simulink model "planta_controlador"  (R2025b)
settings: Solver=FixedStepAuto  StartTime=0.0  StopTime=inf  FixedStep=Ts2  MaxStep=1e-3  RelTol=1e-3
undefined symbols (not defined in the file): ah_max, at_max, bcx, bcy, bh_eq, bhb, bhEb, bhwu, bt, bt_eq, btb, btw, counter_limit, DiscIntNeverNeededParam, g, h_vec_inicial, Hc, ih, is_scanned_vec_inicial, it, Jh_eq, Jt_eq, Kcy, khwu, Ki_h, Ki_t, Kp_h, Kp_t, Ktw, lambda, Lh, Lh0, lh_0, Lt, magnitude, Mc_max, Ms, Mt, N_xt, P_nom, periodo_pulsos, rhd, rtd, tau_hm, tau_tm, Thb_Max, ThEb_Max, Thm_0, Thm_Max, titahm_0, titatm_0, Ts0, Ts1, Ts2, Ttb_Max, Ttm_0, Ttm_Max, vh_0, vh_max_unloaded, vh_nom ... (+20)
libraries: simulink x17, simulink_extras x2, sl3dlib x1, dspnetwork x1
(part 2 of 2)

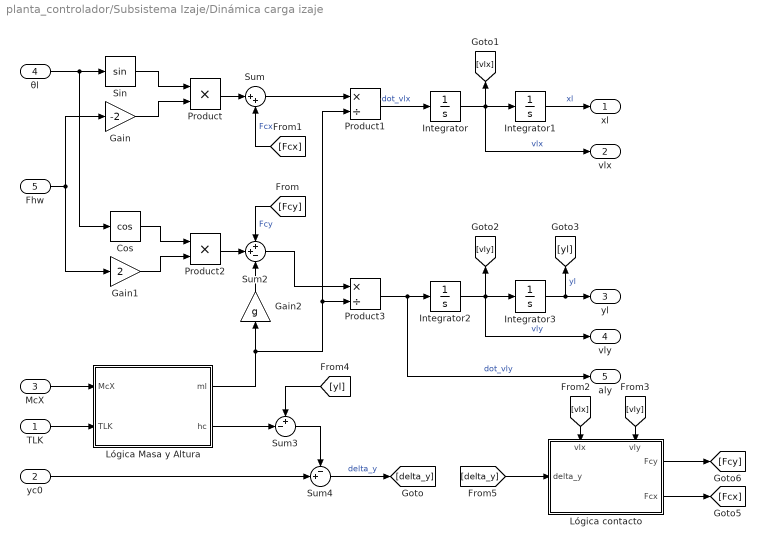
== system planta_controlador/Subsistema Izaje/Dinámica carga izaje ==
  TLK : Inport
  yc0 : Inport  Port=2
  McX : Inport  Port=3
  θl : Inport  Port=4
  Fhw : Inport  Port=5
  Cos : Trigonometry  Operator=cos
  Gain : Gain  Gain=-2
  Gain1 : Gain  Gain=2
  Gain2 : Gain  Gain=g
  Integrator : Integrator  InitialCondition=vlx_0
  Integrator1 : Integrator  InitialCondition=xl_0
  Integrator2 : Integrator  InitialCondition=vly_0
  Integrator3 : Integrator  InitialCondition=yl_0
  Lógica Masa y Altura : Subsystem
  Lógica contacto : Subsystem
      settings: PortSchema="{\"entries\":[{\"content\":{\"sides\":[{\"content\":{\"connectorIds\":[\"In1\"]},\"type\":\"ConnectorPlacement.EquallySpacedRectSide\",\"uuid\":\"20a8b2c4-d5cf-44ce-93ec-929b996a0905\"},{\"content\":{\"connectorIds\":[\"Out1\",\"Out2\"],\"side\":\"RIGHT\"},\"type\":\"ConnectorPlacement.EquallySpacedRectSide\",\"uuid\":\"396e1f2e-cf71-48dc-8d57-a3e2695dfff1\"},{\"content\":{\"connectorIds\":[\"In2\",\"In3\"],\"side\":\"TOP\"},\"type\":\"ConnectorPlacement.EquallySpacedRectSide\",\"uuid\":\"e66c0478-9682-41e1-9b77-d2d789a9c323\"}]},\"type\":\"ConnectorPlacement.EquallySpacedConnector\",\"uuid\":\"193dabd2-f524-433a-b6ef-c1cab585578e\"}],\"packageUris\":[\"http://schema.mathworks.com/mf0/Connector/R2020b\"],\"version\":\"1.0\"}"
  Product : Product
  Product1 : Product  Inputs=*/
  Product2 : Product
  Product3 : Product  Inputs=*/
  Sin : Trigonometry
  Sum : Sum  Inputs=|++
  Sum2 : Sum  Inputs=++-
  Sum3 : Sum  Inputs=+-|
  Sum4 : Sum  Inputs=-+|
  xl : Outport
  vlx : Outport  Port=2
  yl : Outport  Port=3
  vly : Outport  Port=4
  aly : Outport  Port=5
  wires:
  θl/1 -> Sin/1, Cos/1
  Integrator/1 -> vlx/1, Integrator1/1, [vlx]  "vlx"
  Sum3/1 -> Sum4/1
  Sin/1 -> Product/1
  Gain/1 -> Product/2
  [Fcy] -> Sum2/1  "Fcy"
  Integrator2/1 -> vly/1, Integrator3/1, [vly]  "vly"
  Integrator3/1 -> yl/1, [yl]  "yl"
  Fhw/1 -> Gain1/1, Gain/1
  [Fcx] -> Sum/2  "Fcx"
  Product/1 -> Sum/1
  Product1/1 -> Integrator/1  "dot_vlx"
  Gain2/1 -> Sum2/3
  Cos/1 -> Product2/1
  Gain1/1 -> Product2/2
  [yl] -> Sum3/1
  Product2/1 -> Sum2/2
  yc0/1 -> Sum4/2
  Sum2/1 -> Product3/1
  Product3/1 -> aly/1, Integrator2/1  "dot_vly"
  Sum/1 -> Product1/1
  Integrator1/1 -> xl/1  "xl"
  Sum4/1 -> [delta_y]  "delta_y"
  Lógica contacto/1(Fcy) -> [Fcy]
  Lógica contacto/2(Fcx) -> [Fcx]
  Lógica Masa y Altura/1(ml) -> Product1/2, Product3/2, Gain2/1
  McX/1 -> Lógica Masa y Altura/1(McX)
  TLK/1 -> Lógica Masa y Altura/2(TLK)
  Lógica Masa y Altura/2(hc) -> Sum3/2
  [vlx] -> Lógica contacto/2(vlx)
  [vly] -> Lógica contacto/3(vly)
  [delta_y] -> Lógica contacto/1(delta_y)

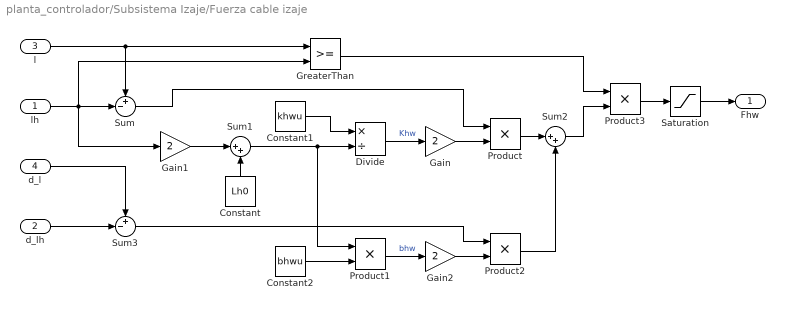
== system planta_controlador/Subsistema Izaje/Fuerza cable izaje ==
  lh : Inport
  d_lh : Inport  Port=2
  l : Inport  Port=3
  d_l : Inport  Port=4
  Constant : Constant  Value=Lh0
  Constant1 : Constant  Value=khwu
  Constant2 : Constant  Value=bhwu
  Divide : Product  Inputs=*/  RndMeth=Zero  SaturateOnIntegerOverflow=on
  Gain : Gain  Gain=2
  Gain1 : Gain  Gain=2
  Gain2 : Gain  Gain=2
  GreaterThan : RelationalOperator  OutDataTypeStr=boolean  RndMeth=Simplest  InputSameDT=off
  Product{,1..3} (4 alike) : Product
  Saturation : Saturate  UpperLimit=inf  LowerLimit=0
  Sum : Sum  Inputs=+-|
  Sum1 : Sum  Inputs=|++
  Sum2 : Sum  Inputs=|++
  Sum3 : Sum  Inputs=+-|
  Fhw : Outport
  wires:
  Constant/1 -> Sum1/2
  Constant2/1 -> Product1/2
  Sum1/1 -> Divide/2, Product1/1
  lh/1 -> Sum/2, GreaterThan/2, Gain1/1
  Product/1 -> Sum2/1
  Gain1/1 -> Sum1/1
  l/1 -> Sum/1, GreaterThan/1
  Product2/1 -> Sum2/2
  Product3/1 -> Saturation/1
  GreaterThan/1 -> Product3/1
  d_lh/1 -> Sum3/2
  Constant1/1 -> Divide/1
  Product1/1 -> Gain2/1  "bhw"
  Sum/1 -> Product/1
  Gain2/1 -> Product2/2
  Divide/1 -> Gain/1  "Khw"
  Sum2/1 -> Product3/2
  Sum3/1 -> Product2/1
  d_l/1 -> Sum3/1
  Gain/1 -> Product/2
  Saturation/1 -> Fhw/1

== system planta_controlador/Subsistema Carro/Accionamiento carro/Freno Motor ==
  BRK_t : Inport
  wtm : Inport  Port=2
  Constant : Constant  Value=0
  Gain3 : Gain  Gain=-Ttb_Max
  Gain4 : Gain  Gain=btb
  Switch : Switch  Criteria=u2 > Threshold  SaturateOnIntegerOverflow=off  InputSameDT=off
  Tanh : Trigonometry  Operator=tanh
  Ttb : Outport
  wires:
  BRK_t/1 -> Switch/2
  Constant/1 -> Switch/1
  wtm/1 -> Gain4/1
  Gain4/1 -> Tanh/1
  Tanh/1 -> Gain3/1
  Gain3/1 -> Switch/3
  Switch/1 -> Ttb/1

== system planta_controlador/Subsistema Izaje/Accionamiento izaje/Freno Emergencia (Drum) ==
  BRK_hE : Inport
  whd : Inport  Port=2
  Constant : Constant  Value=0
  Gain3 : Gain  Gain=-ThEb_Max
  Gain4 : Gain  Gain=bhEb
  Switch : Switch  Criteria=u2 > Threshold  SaturateOnIntegerOverflow=off  InputSameDT=off
  Tanh : Trigonometry  Operator=tanh
  ThEb : Outport
  wires:
  BRK_hE/1 -> Switch/2
  Gain3/1 -> Switch/3
  Constant/1 -> Switch/1
  whd/1 -> Gain4/1
  Gain4/1 -> Tanh/1
  Tanh/1 -> Gain3/1
  Switch/1 -> ThEb/1

== system planta_controlador/Subsistema Izaje/Accionamiento izaje/Freno Motor ==
  BRK_h : Inport
  whm : Inport  Port=2
  Constant : Constant  Value=0
  Gain3 : Gain  Gain=-Thb_Max
  Gain4 : Gain  Gain=bhb
  Switch : Switch  Criteria=u2 > Threshold  SaturateOnIntegerOverflow=off  InputSameDT=off
  Tanh : Trigonometry  Operator=tanh
  Thb : Outport
  wires:
  BRK_h/1 -> Switch/2
  Gain3/1 -> Switch/3
  Constant/1 -> Switch/1
  whm/1 -> Gain4/1
  Gain4/1 -> Tanh/1
  Tanh/1 -> Gain3/1
  Switch/1 -> Thb/1

== system planta_controlador/Subsistema Izaje/Dinámica carga izaje/Lógica Masa y Altura ==
  McX : Inport
  TLK : Inport  Port=2
  Constant : Constant  Value=Ms
  Constant1 : Constant  Value=0
  Constant2 : Constant  Value=Hc
  Rate Limiter : RateLimiter  Commented=through  RisingSlewLimit=Mc_max/0.1  FallingSlewLimit=-Mc_max/0.1  SampleTimeMode=inherited  InitialCondition=Ms
  Sum1 : Sum  Inputs=|++
  Switch : Switch  Criteria=u2 > Threshold  SaturateOnIntegerOverflow=off  InputSameDT=off
  Switch1 : Switch  Criteria=u2 > Threshold  SaturateOnIntegerOverflow=off  InputSameDT=off
  ml : Outport
  hc : Outport  Port=2
  wires:
  Sum1/1 -> Switch/1
  Constant2/1 -> Switch1/1
  TLK/1 -> Switch1/2, Switch/2
  Constant/1 -> Switch/3, Sum1/2
  Constant1/1 -> Switch1/3
  McX/1 -> Sum1/1
  Switch/1 -> Rate Limiter/1
  Rate Limiter/1 -> ml/1
  Switch1/1 -> hc/1

== system planta_controlador/Subsistema Izaje/Dinámica carga izaje/Lógica contacto ==
  delta_y : Inport
  vlx : Inport  Port=2
  vly : Inport  Port=3
  Constant3 : Constant  Value=0
  Constant4 : Constant  Value=0
  Gain3 : Gain  Gain=Kcy
  Gain4 : Gain  Gain=bcy
  Gain5 : Gain  Gain=-bcx
  Saturation : Saturate  UpperLimit=60e5  LowerLimit=0
  Sum5 : Sum  Inputs=-+|
  Switch2 : Switch  SaturateOnIntegerOverflow=off  InputSameDT=off
  Switch3 : Switch  SaturateOnIntegerOverflow=off  InputSameDT=off
  Fcy : Outport
  Fcx : Outport  Port=2
  wires:
  Sum5/1 -> Switch2/1
  vlx/1 -> Gain5/1
  Gain4/1 -> Sum5/1
  vly/1 -> Gain4/1
  Constant4/1 -> Switch3/3
  Gain5/1 -> Switch3/1
  Gain3/1 -> Sum5/2
  delta_y/1 -> Switch3/2, Gain3/1, Switch2/2
  Constant3/1 -> Switch2/3
  Switch2/1 -> Saturation/1  "Fcy"
  Switch3/1 -> Fcx/1  "Fcx"
  Saturation/1 -> Fcy/1

== matlab function planta_controlador/MATLAB Function ==
  data: TLK input; M_carga output; Mc_min parameter
function M_carga = Masa_Aleatoria(TLK, Mc_min)
    persistent masa_actual;
    persistent ultimo_estado_trigger;
    
    % Inicialización
    if isempty(masa_actual)
        masa_actual = Mc_min; % Empezamos con el valor mínimo por defecto
        ultimo_estado_trigger = 0;
    end
    
    % DETECCIÓN DE FLANCO DE SUBIDA (Rising Edge)
    if (TLK == 1 && ultimo_estado_trigger == 0)
        % Generar carga aleatoria entre 3tn y 55tn (para tener sobrecarga)
        masa_actual = Mc_min + (55000 - Mc_min) * rand();
        masa_actual = round(masa_actual); 
    end
    
    % Actualizar memoria del trigger
    ultimo_estado_trigger = TLK;
    % Salida: La masa se mantiene constante hasta el próximo trigger
    M_carga = masa_actual;
end

== stateflow chart planta_controlador/Control Nivel 1 ==
  settings: updateMethod=DISCRETE  sampleTime=Ts1
  state AUTOMATA_PRINCIPAL [parallel]
    entry:
    dead_zone = 0.1; % Zona muerta joystick
    modo_posicion_segura = 0;
    modo_manual_auto = 0;
    seleccionando = 0; ejec_mov = 0;
    is_cont = 0; seleccionando = 0;
    error_der = 0; error_izq = 0;
    error_sup = 0; error_inf = 0;
    error_generic = 0;
    envolvente = zeros(33,1);
    during:
    Joy_CMD_X = Joy_XY(1);
    Joy_CMD_Y = Joy_XY(2);
    settings: executionOrder=1
    state MODO_AUTO
      exit:
      seleccionando_i = [0,0];
      i_obj_vec = [0,0];
      modo_auto = 0;
      modo_manual_auto = 0;
      seleccionando = 0;
      ejec_mov = 0;
      state SELECCION_INDICE_INI
        entry:
        seleccionando_i(1) = 1;
        seleccionando = 1;
        during:
        i_ini = i_x_cruz;
        is_cont = Check_Container(i_ini, yc0_vec);
        exit:
        i_obj_vec(1) = i_ini;
        seleccionando_i(1) = 0;
      state SELECCION_INDICE_FIN
        entry:
        seleccionando_i(2) = 1;
        seleccionando = 1;
        invalido = 0;
        during:
        i_fin = i_x_cruz;
        if (i_fin == 33 || i_fin == 13 || i_fin == 1)
        invalido = 1;
        else invalido = 0; end
        exit:
        i_obj_vec(2) = i_fin;
        seleccionando_i(2) = 0;
      state AUTO_INIT
        entry:
        modo_auto = 1;
        BRK_t_N1 = 1; BRK_h_N1 = 1;
        estado = 1; % Etapa de movimiento
        if (TLK == 1)
        estado = 2;
        i_ini = 0;
        end
        i_obj_vec = [0,0];
        seleccionando_i = [0,0];
      state SELECCION_TRAYECTORIA
        entry:
        modo_auto = 1;
        manual_ok = 0;
        i_usado = 1;
        seleccionando = 0;
        if (estado == 1)
        i_usado = i_ini;
        elseif (estado == 2)
        i_usado = i_fin;
        end
        safe_trajectory = 0; % Asumimos segura
        for k = i_carro:i_usado
        if is_scanned_vec(k) == 0
        safe_trajectory = 1;  % Insegura
        end
        end
      state MOVIMIENTO_CURVO
        entry: ejec_mov = 1;
        during:
        [vx_target, vy_target, manual_ok] = Planificador_Trayectoria_Vel(xt_enc,...
        yh_enc, vt_obs, vh_obs, i_usado, envolvente, TLK, theta_l, vh_lim);
        x_cruz = xt_enc; y_cruz = yh_enc;
        exit: ejec_mov = 0;
      state MODO_MANUAL_SIMPLE
        entry:
        modo_auto = 0;
        modo_manual_auto = 1;
        during:
        if (abs(Joy_CMD_X) < dead_zone)
        vx_target = 0;
        else
        vx_target = Joy_CMD_X * 0.05;
        end
        if (abs(Joy_CMD_Y) < dead_zone)
        vy_target = 0;
        else
        vy_target = Joy_CMD_Y * vh_lim;
        end
        x_cruz = xt_enc; y_cruz = yh_enc;
        exit:
        estado = estado + 1;
        modo_manual_auto = 0;
      state MOVIMIENTO_SEGURO
        entry: ejec_mov = 1;
        during:
        [vx_target, vy_target, manual_ok] = Planificador_Trayectoria_Segura_Vel...
        (xt_enc, yh_enc, vt_obs, i_usado, envolvente, TLK, theta_l, vh_lim);
        x_cruz = xt_enc; y_cruz = yh_enc;
        exit: ejec_mov = 0;
      (default) -> AUTO_INIT
      SELECCION_INDICE_INI -> SELECCION_INDICE_FIN : [BTN_TLK &&...
          |  is_cont == 1]
      (junction 1100) -> SELECCION_INDICE_INI [order 1] : [TLK == 0]
      AUTO_INIT -> (junction 1100)
      (junction 1100) -> SELECCION_INDICE_FIN [order 2] : [TLK == 1]
      SELECCION_INDICE_FIN -> SELECCION_TRAYECTORIA : [BTN_TLK &&...
          |  invalido == 0]
      SELECCION_TRAYECTORIA -> MOVIMIENTO_CURVO [order 2] : [safe_trajectory == 0]
      MOVIMIENTO_CURVO -> (junction 868)
      MODO_MANUAL_SIMPLE -> SELECCION_TRAYECTORIA : [TLK == 1 && yh_enc > (envolvente(i_usado) + Hc) &&...
          |  abs(vh_obs) < 0.1 && estado == 1]
      SELECCION_TRAYECTORIA -> MOVIMIENTO_SEGURO [order 1] : [safe_trajectory == 1]
      (junction 868) -> MODO_MANUAL_SIMPLE : [manual_ok == 1]
      MOVIMIENTO_SEGURO -> (junction 868)
    state STAND_BY
      entry:
      x_cruz_unity = xt_enc; y_cruz_unity = yh_enc;
      modo_standby = 1;
      BRK_t_N1 = 0; BRK_h_N1 = 0; % Frenos Cerrados
      modo_manual = 0; modo_auto = 0;
      modo_error = 0;
      error_der = 0; error_izq = 0;
      error_sup = 0; error_inf = 0;
      error_generic = 0;
      during:
      x_cruz = xt_enc; y_cruz = yh_enc;
      exit:
      modo_standby = 0;
    state ERROR_GENERIC
      entry:
      BRK_t_N1 = 0; BRK_h_N1 = 0;
      modo_error = 1;
      recup_ok = 0;
      error_generic = 1;
    state RECUPERACION
      entry:
      BRK_t_N1 = 1; BRK_h_N1 = 1;
      modo_posicion_segura = 1;
      vel_error = 0.1;
      modo_error = 0;
      during:
      if (abs(Joy_CMD_X) < dead_zone)
      vx_target = 0;
      else
      vx_target = Joy_CMD_X * vt_max/3;
      if (error_der == 1)
      vx_target = Joy_CMD_X * vel_error;
      if (vx_target > 0) vx_target = 0; end
      elseif (error_izq == 1)
      vx_target = Joy_CMD_X * vel_error;
      if (vx_target < 0) vx_target = 0; end
      end
      end
      if (abs(Joy_CMD_Y) < dead_zone)
      vy_target = 0;
      else
      vy_target = Joy_CMD_Y * vh_lim/3;
      if (error_sup == 1)
      vy_target = Joy_CMD_Y * vel_error;
      if (vy_target > 0) vy_target = 0; end
      elseif (error_inf == 1)
      vy_target = Joy_CMD_Y * vel_error;
      if (vy_target < 0) vy_target = 0; end
      end
      end
      x_cruz = xt_enc; y_cruz = yh_enc;
      exit:
      recup_ok = 1;
      modo_posicion_segura = 0;
    state ERROR_INF
      entry:
      BRK_t_N1 = 1; BRK_h_N1 = 0;
      modo_error = 1;
      recup_ok = 0;
      error_inf = 1;
    state PASO_STANDBY
      entry:
      modo_standby = 1;
      during:
      x_cruz = xt_enc;
      y_cruz = yh_enc;
      vx_target = 0; vy_target = 0;
      exit:
      modo_standby = 0;
    state MODO_MANUAL
      entry:
      % Frenos abiertos
      BRK_t_N1 = 1; BRK_h_N1 = 1;
      modo_manual = 1;
      during:
      if (abs(Joy_CMD_X) < dead_zone)
      vx_target = 0;
      else
      vx_target = Joy_CMD_X * vt_max;
      end
      if (abs(Joy_CMD_Y) < dead_zone)
      vy_target = 0;
      else
      vy_target = Joy_CMD_Y * vh_lim;
      end
      x_cruz = xt_enc; y_cruz = yh_enc;
      exit:
      modo_manual = 0;
    state ERROR_SUP
      entry:
      BRK_t_N1 = 1; BRK_h_N1 = 0;
      modo_error = 1;
      recup_ok = 0;
      error_sup = 1;
    state ERROR_IZQ
      entry:
      BRK_t_N1 = 0; BRK_h_N1 = 1;
      modo_error = 1;
      recup_ok = 0;
      error_izq = 1;
    state ERROR_DER
      entry:
      BRK_t_N1 = 0; BRK_h_N1 = 1;
      modo_error = 1;
      recup_ok = 0;
      error_der = 1;
    (default) -> STAND_BY
    STAND_BY -> MODO_AUTO [order 1] : [BTN_Auto &&...
        |  yh_enc >= envolvente(i_carro)]
    MODO_AUTO -> STAND_BY [order 3] : [modo_manual_auto == 1 &&...
        | sobrecarga == 1]
    RECUPERACION -> STAND_BY [order 1] : [BTN_Reset &&...
        |  abs(theta_l) < 0.006 &&...
        |  abs(theta_l_dot) < 0.006 &&...
        |  abs(vt_obs) < 0.01 &&...
        |  abs(vh_obs) < 0.01]
    MODO_AUTO -> STAND_BY [order 4] : [modo_manual_auto == 1 &&...
        |  (TLK == 0 &&...
        |  yh_enc > envolvente(i_usado) &&...
        |  abs(vh_obs) < 0.1 && estado == 2)]
    (junction 1093) -> ERROR_GENERIC [order 5] : [(FALLA_MAN == 1 ||...
        |  FALLA_WD == 1 ||...
        |  FALLA_HSV == 1) &&...
        |  error_generic == 0]
    MODO_MANUAL -> STAND_BY [order 2] : [duration((abs(Joy_XY(1)) < 0.1 &&...
        |  abs(Joy_XY(2)) < 0.1 &&...
        |  abs(vt_obs) < 0.01 &&...
        |  abs(vh_obs) < 0.01 &&...
        |  abs(theta_l_dot) < 0.006 &&...
        |  abs(theta_l) < 0.006), sec) > 1]
    STAND_BY -> MODO_MANUAL [order 2] : [abs(Joy_XY(1)) > dead_zone ||...
        |  abs(Joy_XY(2)) > dead_zone]
    PASO_STANDBY -> STAND_BY [order 1] : [abs(theta_l) < 0.006 &&...
        |  abs(theta_l_dot) < 0.006 &&...
        |  abs(vt_obs) < 0.01 &&...
        |  abs(vh_obs) < 0.01]
    ERROR_GENERIC -> (junction 1295)
    (junction 1093) -> ERROR_INF [order 2] : [(FC_inf == 1 ||...
        |  FALLA_Hinf == 1) &&...
        |  error_inf == 0]
    ERROR_INF -> (junction 1295)
    MODO_AUTO -> PASO_STANDBY [order 7] : [BTN_Reset]
    (junction 1093) -> ERROR_SUP [order 4] : [(FC_sup == 1 ||...
        |  FALLA_Hsup == 1) &&...
        |  error_sup == 0]
    (junction 1295) -> RECUPERACION : [BTN_Reset]
    ERROR_SUP -> (junction 1295)
    PASO_STANDBY -> (junction 1333) [order 2]
    ERROR_IZQ -> (junction 1295)
    ERROR_DER -> (junction 1295)
    (junction 1093) -> ERROR_IZQ [order 3] : [(FC_izq == 1 ||...
        |  FALLA_Tizq == 1) &&...
        |  error_izq == 0]
    MODO_AUTO -> MODO_MANUAL [order 6] : [modo_manual_auto == 1 &&...
        |  abs(Joy_XY(1)) > dead_zone && ...
        |  yh_enc >= envolvente(i_carro) + (TLK * Hc) + 1]
    MODO_AUTO -> MODO_MANUAL [order 5] : [BTN_Manual]
    MODO_AUTO -> MODO_MANUAL [order 1] : [ejec_mov == 1 &&...
        |  (abs(Joy_XY(1)) > dead_zone ||...
        |  abs(Joy_XY(2)) > dead_zone)]
    (junction 1093) -> ERROR_DER [order 1] : [(FC_der == 1 ||...
        |  FALLA_Tder == 1) &&...
        |  error_der == 0]
    MODO_MANUAL -> (junction 1280) [order 1]
    RECUPERACION -> (junction 1093) [order 2]
    (junction 1280) -> (junction 1093)
    (junction 1333) -> (junction 1280)
    MODO_AUTO -> (junction 1333) [order 2]
  state CRUCETA_INDICES_PERFIL [parallel]
    settings: executionOrder=4
    state ACTUALIZAR_CRUCETA [parallel]
      during:
      x_cruz = x_cruz + vx_cmd * Ts1; % Actualizar X cruceta
      y_cruz = y_cruz + vy_cmd * Ts1; % Actualizar Y cruceta
      % Limitar en X
      x_cruz = max(xt_min, min(xt_max, x_cruz));
      % Limitar en Y
      y_cruz = max(yh_min, min(yh_max, y_cruz));
      if seleccionando == 0
      x_cruz_unity = x_cruz;
      y_cruz_unity = y_cruz;
      else
      x_cruz_unity = xt_min + i_x_cruz * Wc - Wc/2;
      y_cruz_unity = yh_min;
      end
      settings: executionOrder=1
    state ACTUALIZAR_PERFIL_ALTURAS [parallel]
      entry:
      yc0_vec = yc0_vec_inicial; yc0 = 0;
      h_vec_output = h_vec_inicial; TLK_anterior = 0;
      is_scanned_vec = is_scanned_vec_inicial;
      during:
      yc0_vec(i_lidar) = h_vec_output(i_lidar); % Actualizo perfil
      is_scanned_vec(i_lidar) = 1;
      % Detecto si se ha abierto o cerrado TLK
      TLK_rise  = (TLK_anterior == 0) && (TLK == 1);
      TLK_fall  = (TLK_anterior == 1) && (TLK == 0);
      if(TLK_rise) % Si agarré un container, hay que bajar el perfil
      h_vec_output(i_carro) = h_vec_output(i_carro) - Hc;
      yc0_vec(i_carro) = yc0_vec(i_carro) - Hc;
      elseif(TLK_fall) % Si solté un container, hay que subir el perfil
      h_vec_output(i_carro) = h_vec_output(i_carro) + Hc;
      yc0_vec(i_carro) = yc0_vec(i_carro) + Hc;
      end
      TLK_anterior = TLK; yc0 = yc0_vec(i_carro);
      envolvente = Generar_Envolvente(yc0_vec, is_scanned_vec);
      settings: executionOrder=2
    state CALCULO_INDICES [parallel]
      entry:
      i_carro = 1; i_lidar = 1; i_x_cruz = 1;
      during:
      i_carro = floor((xt_enc - xt_min)/Wc) + 1;
      i_carro = min(max(i_carro, 1), 33);
      i_lidar = floor((xt_enc+x_LIDAR-xt_min)/Wc)+1;
      i_lidar = min(max(i_lidar,1),33);
      i_x_cruz = floor((x_cruz - xt_min)/Wc) + 1;
      i_x_cruz = min(max(i_x_cruz, 1), 33);
      settings: executionOrder=3
  state LIMITES_SUAVES [parallel]
    entry: K_acc = 0.65;
    during:
    % LÍMITE INFERIOR DE IZAJE
    if (TLK == 1)
    dist = yh_enc - (yc0 + 0.5 + Hc); T_retardo = 0.8;
    else
    dist = yh_enc - (yc0 + 0.5); T_retardo = 0.4;
    end
    % Compensación con retardo dinámico
    dist_efectiva = dist - (abs(vy_cmd) * T_retardo);
    if (dist_efectiva < 0)
    dist_efectiva = 0;
    end
    acc_plan = ah_max * K_acc;
    v_segura = sqrt(0.01 + 2 * acc_plan * dist_efectiva);
    if (v_segura > vh_lim)
    v_segura = vh_lim;
    end
    % Si pide moverse más rápido, se recorta
    if (vy_cmd < -v_segura)
    vy_cmd = -v_segura;
    end
    % LÍMITE SUPERIOR DE IZAJE
    dist = (yh_max - 2) - yh_enc;
    dist_efectiva = dist - (abs(vy_cmd) * T_retardo);
    if (dist_efectiva < 0)
    dist_efectiva = 0;
    end
    v_segura = sqrt(0.01 + 2 * acc_plan * dist_efectiva);
    if (v_segura > vh_lim)
    v_segura = vh_lim;
    end
    if (vy_cmd > v_segura)
    vy_cmd = v_segura;
    end
    % LÍMITE DERECHO DEL CARRO
    T_retardo = 5; % Retardo mayor para el carro
    dist = (xt_max - 2) - xt_enc;
    dist_efectiva = dist - (abs(vx_cmd) * T_retardo);
    if (dist_efectiva < 0)
    dist_efectiva = 0;
    end
    acc_plan = at_max * K_acc;
    v_segura = sqrt(0.01 + 2 * acc_plan * dist_efectiva);
    if (vx_cmd > v_segura)
    vx_cmd = v_segura;
    end
    % LÍMITE IZQUIERDO DEL CARRO
    dist = xt_enc - (xt_min + 2);
    dist_efectiva = dist - (abs(vx_cmd) * T_retardo);
    if (dist_efectiva < 0)
    dist_efectiva = 0;
    end
    v_segura = sqrt(0.01 + 2 * acc_plan * dist_efectiva);
    if (vx_cmd < -v_segura)
    vx_cmd = -v_segura;
    end
    settings: executionOrder=5
  state TWISTLOCKS [parallel]
    settings: executionOrder=2
    state CARGADO
      entry:
      m_container = m_est - Ms; % Masa estimada container
      if (m_container > (Mc_max + 100)) % Margen de 100kg
      sobrecarga = 1;
      end
      during:
      m_est = max(Ms, (Fhw * 2 / g));
      vh_lim = min(vh_max_unloaded,...
      max(vh_nom, P_nom / ((m_container + Ms) * g)));
      if (sobrecarga == 1)
      vh_lim = 0.1; vx_target = 0;
      if (vy_target > 0) vy_target = 0; end
      end
    state CERRANDO_TLK
      entry:
      TLK = 1;
      y_start = yh_enc;
      m_est = max(Ms, (Fhw * 2 / g));
      during:
      vh_lim = 0.1;
      vx_target = 0;
      % Filtro simple
      m_est = m_est + 0.1 *...
      (max(Ms, (Fhw * 2 / g)) - m_est);
    state ABRIENDO_TLK
      entry:
      TLK = 0;
      y_start = yh_enc;
      m_container = 0;
      sobrecarga = 0;
      during:
      m_est = max(Ms, Fhw * 2 / g);
      vh_lim = 0.1;
      vx_target = 0;
    state VACIO
      entry:
      TLK = 0;
      m_est = Ms;
      sobrecarga = 0;
      during:
      hay_cont = Check_Container...
      (i_carro, yc0_vec);
      vh_lim = vh_max_unloaded;
    (default) -> VACIO
    CERRANDO_TLK -> CARGADO : [Fhw > (Ms*g/2 * 1.2) &&...
        |  abs(yh_enc - y_start) > 0.3 &&...
        |  abs(vt_obs) < 0.01]
    VACIO -> CERRANDO_TLK : [BTN_TLK == 1 &&...
        |  Fhw < (Ms*g/2 * 0.8) &&...
        |  hay_cont == 1]
    CARGADO -> ABRIENDO_TLK : [BTN_TLK == 1 &&...
        |  Fhw < ((m_est*g/2)*0.8) &&...
        | ~ismember(i_carro, [1, 13, 33])]
    ABRIENDO_TLK -> VACIO : [Fhw > (Ms*g/2*0.8) && abs(yh_enc - y_start) > 0.3 && abs(vt_obs) < 0.01]
  state SUAVIZADO_VELOCIDAD [parallel]
    entry:
    ax_act = 0; ay_act = 0;
    jerk_max = 1.5; v_max_ref = 12;
    vx_cmd = 0; vy_cmd = 0;
    vx_target = 0; vy_target = 0;
    during:
    if (seleccionando == 1)
    vx_target = Joy_CMD_X * v_max_ref;
    vx_cmd = vx_target;
    else
    [vx_cmd, ax_act] = Suavizador_Cinematico...
    (vx_target, vx_cmd, ax_act, at_max, jerk_max);
    [vy_cmd, ay_act] = Suavizador_Cinematico...
    (vy_target, vy_cmd, ay_act, ah_max, jerk_max);
    end
    settings: executionOrder=3
  state WATCHDOG_HEARTBEAT [parallel]
    settings: executionOrder=6
    state PULSOS_UP
      entry:
      heartbeat = 0;
    state PULSOS_DOWN
      entry:
      heartbeat = 1;
    (default) -> PULSOS_UP
    PULSOS_DOWN -> PULSOS_UP : [after(periodo_pulsos, msec)]
    PULSOS_UP -> PULSOS_DOWN : [after(periodo_pulsos, msec)]
  data: i_pos function_input; y0_vec function_input; hay_container function_output; v_target function_input; v_act function_input; a_act function_input; A_MAX function_input; J_MAX function_input; v_out function_output; a_out function_output; perfil_escaneado_vec function_input; escaneado_vec function_input; envolvente_f function_output; x_real function_input; y_real function_input; vx_carro function_input; vy_izaje function_input; i_ref function_input; envolvente_vec function_input; twistlock function_input; tita_l function_input; vh_limit function_input; vx_ref function_output; vy_ref function_output; listo function_output; x_real function_input; y_real function_input; vx_carro function_input; i_ref function_input; envolvente_vec function_input; twistlock function_input; tita_l function_input; vh_limit function_input; vx_ref function_output; vy_ref function_output; listo function_output; theta_l_dot input; vt_obs input; Fhw input size=1; BTN_TLK input size=1; m_est output size=1; vh_lim output size=1; Joy_XY input; BTN_Manual input size=1; BTN_Auto input size=1; BTN_Reset input size=1; FC_der input size=1; FC_sup input size=1; FC_izq input size=1; FC_inf input size=1; yh_enc input size=1; vh_obs input; BRK_h_N1 output size=1; BRK_t_N1 output size=1; TLK output size=1; h_vec_output output; modo_manual output; modo_auto output; theta_l input; seleccionando_i output; i_obj_vec output; x_cruz_unity output; y_cruz_unity output; modo_posicion_segura output; modo_error output; modo_manual_auto output; modo_standby output; ejec_mov output; sobrecarga output; m_container output; heartbeat output; recup_ok output; vx_cmd output; envolvente output; vy_cmd output; xt_enc input; dead_zone local; manual_ok local; is_scanned_vec local; safe_trajectory local; v_max_ref local; Joy_CMD_X local; Joy_CMD_Y local; vy_target local; vx_target local; T_retardo local; dist_efectiva local; TLK_anterior local; estado local; i_ini local; is_cont local; i_x_cruz local; yc0_vec local; invalido local; i_fin local; x_cruz local; y_cruz local; i_usado local; i_carro local; k local; ax_act local; ay_act local; jerk_max local; K_acc local; y_start local; dist local; yc0 local; v_segura local; acc_plan local; i_lidar local; TLK_fall local; TLK_rise local; vh_max_unloaded parameter; vt_max parameter; Ts1 parameter; at_max parameter; ah_max parameter; yh_min parameter; yh_max parameter; Wc parameter; x_LIDAR parameter; Hc parameter; is_scanned_vec_inicial parameter; yc0_vec_inicial parameter; g parameter; Ms parameter; P_nom parameter; Mc_max parameter; vh_nom parameter; xt_max parameter; xt_min parameter; N_xt parameter; periodo_pulsos parameter; h_vec_inicial parameter; hay_cont local; seleccionando output; FALLA_Tizq input; FALLA_Tder input; FALLA_HSV input; FALLA_Hsup input; FALLA_Hinf input; FALLA_WD input; FALLA_MAN input; error_generic local; vel_error local; error_inf output; error_der output; error_izq output; error_sup output; Yt0 parameter
  function hay_container = Check_Container(...:
    | function hay_container = Check_Container(...
    |     i_pos, y0_vec)
    | 
    | if(i_pos<13 && y0_vec(i_pos)>0)
    |    hay_container = 1;
    | elseif(i_pos>13 && i_pos<33 && y0_vec(i_pos)>-18)
    |    hay_container = 1;
    | else
    |    hay_container = 0;
    | end
    | 
    | end
  function [v_out, a_out] = Suavizador_Cinematico...:
    | function [v_out, a_out] = Suavizador_Cinematico...
    |     (v_target, v_act, a_act, A_MAX, J_MAX)
    | 
    | err_v = v_target - v_act;   % Error instantáneo de velocidad    
    | zona_lineal = 0.05;         % Zona lineal cercana a cero para evitar singularidad en la raíz
    | 
    | %% Generación de aceleración deseada
    | if abs(err_v) < 1e-6        % Evita micro-oscilaciones cuando el error es prácticamente cero.
    |     v_out = v_target;
    |     a_out = 0;
    |     return;
    | % Ley tipo raíz cuadrada
    | elseif abs(err_v) > zona_lineal        
    |     a_req = sign(err_v) * sqrt(2 * J_MAX * abs(err_v)); % Región no lineal
    | else
    |     a_req = (err_v / zona_lineal) * sqrt(2 * J_MAX * zona_lineal);  % Región lineal cercana a cero para evitar pendiente infinita
    | end
    | 
    | %% Saturación de aceleración
    | if a_req > A_MAX
    |     a_req = A_MAX;
    | elseif a_req < -A_MAX
    |     a_req = -A_MAX;
    | end
    | 
    | %% Cálculo de jerk requerido
    | jerk_req = (a_req - a_act) / Ts1;
    | % Saturación de jerk
    | if jerk_req > J_MAX
    |     jerk_req = J_MAX;
    | elseif jerk_req < -J_MAX
    |     jerk_req = -J_MAX;
    | end
    | 
    | %% Integración discreta (Euler)
    | a_out = a_act + jerk_req * Ts1;
    | v_out = v_act + a_out * Ts1;
    | 
    | %% Eliminación de deriva
    | % Forzar a cero absoluto si el joystick está suelto
    | if abs(v_target) < 0.001 && abs(v_out) < 0.001
    |     v_out = 0.0;
    |     a_out = 0.0;
    | end
    | 
    | end
  function envolvente_f = Generar_Envolvente...:
    | function envolvente_f = Generar_Envolvente...
    |     (perfil_escaneado_vec, escaneado_vec)
    | 
    | N = 33; % No puedo usar N_xt, da error
    | h_seguridad = Hc/2; % Margen fijo (ajustable)
    | 
    | perfil_seguro = zeros(N,1);
    | for i = 1:N
    |     if escaneado_vec(i) == 1
    |         perfil_seguro(i) = perfil_escaneado_vec(i) + h_seguridad;
    |     else
    |         perfil_seguro(i) = 0;
    |     end
    | end
    | 
    | envolvente_f = perfil_seguro;
    | 
    | for i = 1:N
    |     if escaneado_vec(i) == 0
    |         continue;
    |     end
    | 
    |     e_i = perfil_seguro(i);
    |     % vecino izquierdo
    |     if i > 1 && escaneado_vec(i-1) == 1
    |         if e_i > perfil_seguro(i-1)
    |             envolvente_f(i-1) = max(envolvente_f(i-1), e_i);
    |         end
    |     end
    |     % vecino derecho
    |     if i < N && escaneado_vec(i+1) == 1
    |         if e_i > perfil_seguro(i+1)
    |             envolvente_f(i+1) = max(envolvente_f(i+1), e_i);
    |         end
    |     end
    | end
    | 
    | for i = 1:N
    |     if escaneado_vec(i) == 0
    |         envolvente_f(i) = 0;
    |     end
    | end
    | 
    | end
  function [vx_ref, vy_ref, listo] = Planificador_Trayectoria_Vel(x_real, y_real,...:
    | function [vx_ref, vy_ref, listo] = Planificador_Trayectoria_Vel(x_real, y_real,...
    |     vx_carro, vy_izaje, i_ref, envolvente_vec, twistlock, tita_l, vh_limit)
    | 
    | %% 1. INICIALIZACIÓN
    | persistent last_i_ref
    | if isempty(last_i_ref)
    |     last_i_ref = -1;
    | end
    | if i_ref ~= last_i_ref
    |     last_i_ref = i_ref;
    | end
    | 
    | %% 2. PARÁMETROS GLOBALES FÍSICOS
    | Kp_x = 0.20;  
    | Kd_x = 0.15;
    | Kp_y = 0.38;
    | Kd_y = 0.25;
    | 
    | H_extra = double(twistlock == 1) * Hc;
    | 
    | %% 3. MAPEO DE LA RUTA Y OBSTÁCULOS
    | i_obj = min(max(i_ref, 1), N_xt);
    | i_act = min(max(floor((x_real - xt_min) / Wc) + 1, 1), N_xt);
    | x_dest = xt_min + (i_obj - 0.5) * Wc;
    | 
    | step = sign(i_obj - i_act);
    | if step == 0; step = 1; end
    | 
    | h_obst_fwd = 0;
    | for k = i_act : step : i_obj
    |     if envolvente_vec(k) > h_obst_fwd
    |         h_obst_fwd = envolvente_vec(k);
    |     end
    | end
    | y_techo_ruta = h_obst_fwd + H_extra;
    | 
    | %% 4. SINCRONIZACIÓN CINEMÁTICA
    | % Escaneamos las columnas por delante para ver cuánto tiempo necesitamos para subir
    | limite_vx_sinc = vt_max;
    | 
    | for k = i_act : step : i_obj
    |     techo_seguro = envolvente_vec(k) + H_extra;
    |     dy = techo_seguro - y_real;
    |     
    |     if dy > 0  % Si esa columna está más alta que mi posición actual
    |         xc = xt_min + (k - 0.5) * Wc;
    |         
    |         % Distancia horizontal hasta la "pared" de esa celda
    |         dx = abs(xc - x_real) - (Wc / 2); 
    |         dx = max(0.01, dx); % Evitamos división por cero si estamos muy pegados
    |         
    |         % Tiempo que nos tomará subir ese 'dy' yendo a velocidad de izaje
    |         tiempo_para_subir = dy / vh_limit;
    |         
    |         % La velocidad en X permitida para que nos dé el tiempo de subir sin chocar
    |         vx_max_permitida = (dx + 1.5) / tiempo_para_subir;
    |         
    |         % Nos quedamos siempre con el límite más restrictivo de todo el camino
    |         if vx_max_permitida < limite_vx_sinc
    |             limite_vx_sinc = vx_max_permitida;
    |         end
    |     end
    | end
    | 
    | % Mantenemos una velocidad mínima de 0.10 m/s para que nunca se congele
    | limite_vx_final = max(0.10, min(vt_max, limite_vx_sinc));
    | 
    | % Control PD para el carro
    | l = Yt0 - y_real;  
    | x_carga   = x_real + l * sin(tita_l);
    | e_x   = x_dest - x_carga;
    | vx_req = Kp_x * e_x - Kd_x * vx_carro;
    | 
    | % Saturamos la referencia con nuestro nuevo límite inteligente
    | vx_ref = max(-limite_vx_final, min(limite_vx_final, vx_req));
    | 
    | %% 5. PLANIFICACIÓN VERTICAL EN Y
    | h_dest_final = envolvente_vec(i_obj) + H_extra;
    | 
    | if abs(x_real - x_dest) < (Wc * 0.4)
    |     y_target = h_dest_final;
    | else
    |     y_target = max(h_dest_final, y_techo_ruta + 1);
    | end
    | 
    | % Control PD para el izaje
    | vy_req = Kp_y * (y_target - y_real) - Kd_y * vy_izaje;
    | vy_ref = max(-vh_limit, min(vh_limit, vy_req));
    | 
    | %% 6. SEÑAL DE LISTO
    | listo = double( ...
    |     abs(x_real - x_dest) < 0.05 && ...          
    |     abs(y_real - h_dest_final) < 0.1 && ...     
    |     abs(tita_l) < 0.0174 && ...                 
    |     abs(vx_carro) < 0.05 &&...
    |     abs(vy_izaje) < 0.05);                    
    | end
  function [vx_ref, vy_ref, listo] = Planificador_Trayectoria_Segura_Vel(x_real,...:
    | function [vx_ref, vy_ref, listo] = Planificador_Trayectoria_Segura_Vel(x_real,...
    |     y_real, vx_carro, i_ref, envolvente_vec, twistlock, tita_l, vh_limit)
    | 
    | %% 1. MEMORIA DE LA MÁQUINA DE ESTADOS
    | persistent fase last_i_ref
    | if isempty(fase)
    |     fase = uint8(1);
    |     last_i_ref = -1;
    | end
    | if i_ref ~= last_i_ref
    |     fase = uint8(1);
    |     last_i_ref = i_ref;
    | end
    | 
    | %% 2. PARÁMETROS
    | DIST_X = 1.0;           % Arranca a bajar cuando está a 1m de la celda
    | DIST_Y = 15.0;          % Arranca a cruzar cuando está a 15m del techo de crucero
    | Y_CRUCERO_MIN = 39.0;
    | 
    | Kp_x = 0.20;             
    | Kp_y = 0.38;             
    | 
    | H_extra = double(twistlock == 1) * Hc;
    | 
    | %% 3. ÍNDICES Y DESTINO
    | i_obj = min(max(i_ref, 1), N_xt);
    | i_act = min(max(floor((x_real - xt_min) / Wc) + 1, 1), N_xt);
    | x_dest = xt_min + (i_obj - 0.5) * Wc;
    | h_dest = envolvente_vec(i_obj);
    | y_base = h_dest + H_extra;
    | 
    | % Altura de crucero
    | i_min_ruta = min(i_act, i_obj);
    | i_max_ruta = max(i_act, i_obj);
    | h_max_ruta = max(envolvente_vec(i_min_ruta:i_max_ruta));
    | y_crucero = max(Y_CRUCERO_MIN, h_max_ruta + H_extra);
    | 
    | %% 4. MÁQUINA DE ESTADOS
    | listo = 0;
    | 
    | switch fase
    |     case 1  % SUBIR A CRUCERO
    |         vy_req = Kp_y * (y_crucero - y_real);
    |         vx_req = 0;
    |         
    |         % Transición: Si estamos a menos de DIST_Y del techo, arranca el cruce
    |         if abs(y_real - y_crucero) < DIST_Y 
    |             fase = uint8(2);
    |         end
    |         
    |     case 2  % CRUZAR EN X
    |         % Mantenemos a 'Y' persiguiendo el crucero para que termine de llegar y se quede ahí
    |         vy_req = Kp_y * (y_crucero - y_real); 
    |         vx_req = Kp_x * (x_dest - x_real);
    |         
    |         % Transición: Si el carro llegó (margen DIST_X) y no hay balanceo, empezamos a bajar
    |         if abs(x_real - x_dest) < DIST_X && abs(tita_l) < 0.0175
    |             fase = uint8(3);
    |         end
    |         
    |     case 3  % BAJAR A DESTINO
    |         % Mantenemos a 'X' clavado en el destino
    |         vx_req = Kp_x * (x_dest - x_real);
    |         vy_req = Kp_y * (y_base - y_real);
    |         
    |         % Transición: Llegó al piso y el péndulo está calmado
    |         if abs(y_real - y_base) < 0.1 && abs(tita_l) < 0.0175
    |             fase = uint8(4);
    |         end
    |         
    |     otherwise % FASE 4: LISTO
    |         vx_req = Kp_x * (x_dest - x_real);
    |         vy_req = Kp_y * (y_base - y_real);
    |         listo = double( ...
    |             abs(x_real - x_dest) < 0.05 && ...
    |             abs(y_real - y_base) < 0.1 && ...
    |             abs(tita_l) < 0.0175 && ...
    |             abs(vx_carro) < 0.05);
    | end
    | 
    | %% 5. SATURACIÓN FÍSICA Y SALIDA
    | vx_ref = max(-vt_max, min(vt_max, vx_req));
    | vy_ref = max(-vh_limit, min(vh_limit, vy_req));
    | 
    | end

== stateflow chart planta_controlador/Control Nivel 0 ==
  state ESTADOS_SEGURIDAD [parallel]
    entry:
    vh_lim = vh_max_unloaded;
    settings: executionOrder=1
    state SISTEMA_OK
      entry:
      BRK_hE_N0 = 1; BRK_t_N0 = 1;
      FALLA_MAN = 0; FALLA_WD = 0;
      FALLA_IZAJE_SUP = 0; FALLA_IZAJE_INF = 0;
      FALLA_IZAJE_SV = 0;
      FALLA_CARRO_DER = 0; FALLA_CARRO_IZQ = 0;
      during:
      vh_lim = min(vh_max_unloaded,...
      max(vh_nom, (P_nom / ((m_container+Ms) * g))));
    state EMERGENCIA_CARRO_DER
      entry:
      BRK_hE_N0 = 1; BRK_t_N0 = 0;
      FALLA_CARRO_DER = 1;
    state EMERGENCIA_IZAJE_INF
      entry:
      BRK_hE_N0 = 0; BRK_t_N0 = 1;
      FALLA_IZAJE_INF = 1;
    state EMERGENCIA_IZAJE_SUP
      entry:
      BRK_hE_N0 = 0; BRK_t_N0 = 1;
      FALLA_IZAJE_SUP = 1;
    state EMERGENCIA_MANUAL
      entry:
      BRK_hE_N0 = 0; BRK_t_N0 = 0;
      FALLA_MAN = 1;
    state EMERGENCIA_WD
      entry:
      BRK_hE_N0 = 0; BRK_t_N0 = 0;
    state MODO_RECUPERACION
      entry:
      BRK_hE_N0 = 1; BRK_t_N0 = 1;
      FALLA_MAN = 0;
      FALLA_IZAJE_SV = 0;
    state EMERGENCIA_IZAJE_SV
      entry:
      BRK_hE_N0 = 0; BRK_t_N0 = 1;
      FALLA_IZAJE_SV = 1;
    state EMERGENCIA_CARRO_IZQ
      entry:
      BRK_hE_N0 = 1; BRK_t_N0 = 0;
      FALLA_CARRO_IZQ = 1;
    (default) -> SISTEMA_OK
    EMERGENCIA_CARRO_DER -> (junction 150)
    (junction 144) -> EMERGENCIA_CARRO_DER [order 2] : [FCE_der == 1]
    (junction 120) -> EMERGENCIA_IZAJE_INF [order 2] : [FCE_inf == 1]
    EMERGENCIA_IZAJE_INF -> (junction 138)
    SISTEMA_OK -> (junction 144) [order 1]
    (junction 120) -> EMERGENCIA_IZAJE_SUP [order 1] : [FCE_sup == 1]
    SISTEMA_OK -> (junction 120) [order 3]
    (junction 144) -> EMERGENCIA_CARRO_IZQ [order 1] : [FCE_izq == 1]
    (junction 120) -> EMERGENCIA_IZAJE_SV [order 3] : [abs(vh_obs) > (1.15 * vh_lim)]
    SISTEMA_OK -> EMERGENCIA_WD [order 4] : [FALLA_WD==1]
    MODO_RECUPERACION -> SISTEMA_OK : [recup_ok == 1]
    SISTEMA_OK -> EMERGENCIA_MANUAL [order 2] : [BTN_Emerg]
    EMERGENCIA_IZAJE_SUP -> (junction 138)
    EMERGENCIA_WD -> MODO_RECUPERACION : [BTN_Reset]
    EMERGENCIA_MANUAL -> MODO_RECUPERACION : [BTN_Reset]
    (junction 150) -> MODO_RECUPERACION : [BTN_Reset]
    EMERGENCIA_CARRO_IZQ -> (junction 150)
    EMERGENCIA_IZAJE_SV -> (junction 138)
    (junction 138) -> MODO_RECUPERACION : [BTN_Reset]
  state WATCHDOG [parallel]
    settings: executionOrder=2
    state HEARTBEAT_DOWN
      entry:
      WD_counter = 0;
      during:
      WD_counter = WD_counter + 1;
    state DETECCION_FALLO
      entry:
      FALLA_WD = 1;
    state HEARTBEAT_UP
      entry:
      WD_counter = 0;
      during:
      WD_counter = WD_counter + 1;
    (default) -> HEARTBEAT_DOWN
    HEARTBEAT_DOWN -> DETECCION_FALLO [order 2] : [WD_counter >= counter_limit]
    HEARTBEAT_UP -> HEARTBEAT_DOWN [order 1] : [heartbeat==0]
    HEARTBEAT_DOWN -> HEARTBEAT_UP [order 1] : [heartbeat==1]
    DETECCION_FALLO -> HEARTBEAT_DOWN : [FALLA_WD==0]
    HEARTBEAT_UP -> DETECCION_FALLO [order 2] : [WD_counter >= counter_limit]
  data: BTN_Emerg input size=1; FCE_der input size=1; FCE_sup input size=1; vh_obs input size=1; FCE_izq input size=1; FCE_inf input size=1; BRK_hE_N0 output size=1; BRK_t_N0 output size=1; vh_max_unloaded parameter size=1; BTN_Reset input; FALLA_MAN output; heartbeat input; FALLA_WD output; WD_counter local; m_container input; vh_lim local; recup_ok input; vh_nom parameter; P_nom parameter; g parameter; Ms parameter; counter_limit parameter; FALLA_CARRO_IZQ output; FALLA_IZAJE_SV output; FALLA_IZAJE_SUP output; FALLA_IZAJE_INF output; FALLA_CARRO_DER output

== matlab function planta_controlador/MATLAB Function1 ==
  data: yc0 output; xl input; xt_min parameter; Wc parameter; h_vec input
function yc0 = Y_spreader(xl, xt_min, Wc, h_vec)
% Cálculo índice de spreader
i_spreader = floor((xl - xt_min)/Wc) + 1;
i_spreader = min(max(i_spreader, 1), 33);

% Obtención de yc0 usando la posición del spreader
yc0 = h_vec(i_spreader);

== matlab function planta_controlador/Controlador Carro2/Controlador de Balanceo ==
  data: tita_l input; v_sway output; yh_enc input; anti_sway input; Yt0 parameter; g parameter; lambda parameter
function v_sway = ControlBalanceo(tita_l, yh_enc, anti_sway, Yt0, g, lambda)

lh = abs(Yt0 - yh_enc);

K_sway = 2 *lambda * sqrt(g*lh);

if(anti_sway)
    v_sway = K_sway * tita_l;
else
    v_sway = 0;
end

== matlab function planta_controlador/Controlador Carro2/Modulación de la Referencia ==
  data: vx_cmd input; seleccion input; vt_ref output; v_sway input; Ts2 parameter; at_max parameter; vt_max parameter; vt_0 parameter
function vt_ref = ModulacionRef(vx_cmd, seleccion, v_sway, Ts2, at_max, vt_max, vt_0)

persistent vt_ref_prev

if isempty(vt_ref_prev)
    vt_ref_prev = vt_0;
end

if seleccion > 0
    vel_base = 0;
else
    vel_base = vx_cmd;
end

vt_cmd = vel_base + v_sway;
vt_cmd_sat = min(max(vt_cmd, -vt_max), vt_max);

delta_v = vt_cmd_sat - vt_ref_prev;
limite_delta = at_max * Ts2;
delta_v_limitado = min(max(delta_v, -limite_delta), limite_delta);

vt_ref = vt_ref_prev + delta_v_limitado;
vt_ref_prev = vt_ref;

== matlab function planta_controlador/Controlador Carro2/Observador de Estado ==
  data: xtd_enc input; vt_obs output; Ttm_ref input; wtm_0 parameter; titatm_0 parameter; Lt parameter; bt_eq parameter; Jt_eq parameter; rtd parameter; it parameter; Ts2 parameter
function vt_obs = Observador_Estado_t(xtd_enc, Ttm_ref, wtm_0, titatm_0, Lt, bt_eq, Jt_eq, rtd, it, Ts2)...
    
    % Memorias
    persistent theta_t_obs_prev wt_obs_prev int_e_prev
    
    % Condiciones iniciales
    if isempty(theta_t_obs_prev)
        theta_t_obs_prev = titatm_0;
        wt_obs_prev      = wtm_0;    
        int_e_prev       = 0.0; 
    end
    
    % 1. Convertir posición lineal del carro a angular del motor
    theta_t_enc = xtd_enc * (it / rtd);
    
    % 2. Error de estimación (Posición real vs observada)
    e_theta_t = theta_t_enc - theta_t_obs_prev;
    
    % 3. Lazo de torque (Física de la planta)
    Torque_net = Ttm_ref - (bt_eq * wt_obs_prev) + (Lt(3) * int_e_prev);
    alpha_phys = Torque_net / Jt_eq; % Aceleración angular
    
    % 4. Derivadas
    dot_wt_obs      = alpha_phys + (Lt(2) * e_theta_t);
    dot_theta_t_obs = wt_obs_prev + (Lt(1) * e_theta_t);

    % 5. Salida del observador
    vt_obs = wt_obs_prev * (rtd / it);
    
    % 6. Integración Discreta
    theta_t_obs = theta_t_obs_prev + (Ts2 * dot_theta_t_obs);
    wt_obs      = wt_obs_prev      + (Ts2 * dot_wt_obs);
    int_e       = int_e_prev       + (Ts2 * e_theta_t);

    % 7. Actualizar memorias para el siguiente ciclo de reloj
    theta_t_obs_prev = theta_t_obs;
    wt_obs_prev      = wt_obs;
    int_e_prev       = int_e;
end

== matlab function planta_controlador/Controlador Carro2/Controlador de Velocidad ==
  data: vt_ref input; Ttm_ref output; vt_obs input; BRK_t input; Ts2 parameter; Ki_t parameter; Kp_t parameter
function Ttm_ref = ControlVelocidad(vt_ref, vt_obs, BRK_t, Ts2, Ki_t, Kp_t)
    % Memorias para el integrador
    persistent int_prev e_v_prev
    
    % Inicialización
    if isempty(int_prev)
        int_prev = 0.0;
        e_v_prev = 0.0;
    end
    
    % 1. Cálculo del error de velocidad
    e_v = vt_ref - vt_obs;
    
    % 2. Integrador Discreto (Tustin) con Reset por Freno
    % Si el freno está activo (BRK_t = 0), forzamos la memoria a 0 
    % para evitar la acumulación de error (Anti-Windup).
    if BRK_t > 0
        int_val = int_prev + (Ts2 / 2) * (e_v + e_v_prev);
    else
        int_val = 0.0;
    end
    
    % 3. Controlador PI
    P_out = e_v * Kp_t;
    I_out = int_val * Ki_t;
    
    % Suma final de referencia de torque
    Ttm_ref = P_out + I_out;
    
    % 4. Actualizar memorias
    int_prev = int_val;
    e_v_prev = e_v;
end

== matlab function planta_controlador/Controlador Izaje2/Modulación de la Referencia ==
  data: vy_cmd input; vh_ref output; seleccion input; ah_max parameter; Ts2 parameter; vh_0 parameter; vh_lim input
function vh_ref = ModulacionReferencia(vy_cmd, seleccion, ah_max, Ts2, vh_0, vh_lim)
persistent vh_ref_prev

if isempty(vh_ref_prev)
    vh_ref_prev = vh_0;
end

if seleccion > 0
    vh_cmd = 0;
else
    vh_cmd = vy_cmd;
end

vh_cmd_sat = min(max(vh_cmd, -vh_lim), vh_lim);

delta_v = vh_cmd_sat - vh_ref_prev;
limite_delta = ah_max * Ts2;
delta_v_limitado = min(max(delta_v, -limite_delta), limite_delta);

vh_ref = vh_ref_prev + delta_v_limitado;
vh_ref_prev = vh_ref;
end

== matlab function planta_controlador/Controlador Izaje2/Controlador de Velocidad ==
  data: m_est input; Thm_ref output; vh_ref input; vh_obs input; BRK input; ih parameter; rhd parameter; g parameter; Kp_h parameter; Ki_h parameter; Ts2 parameter
function Thm_ref = ControlVelocidad(m_est, vh_ref, vh_obs, BRK, ih, rhd, g, Kp_h, Ki_h, Ts2)
persistent int_prev e_w_prev

if isempty(int_prev)
    int_prev = 0.0;
    e_w_prev = 0.0;
end

e_w = (vh_ref - vh_obs) * (2 * ih / rhd);

if BRK > 0
    int_val = int_prev + (Ts2 / 2) * (e_w + e_w_prev);
else
    int_val = 0.0;
    e_w_prev = 0.0;
end

T_PID = Kp_h * e_w + Ki_h * int_val;
Tg_ff = m_est * (g * rhd / (2 * ih));

Thm_ref = T_PID + Tg_ff;

int_prev = int_val;
e_w_prev = e_w;
end

== matlab function planta_controlador/Controlador Izaje2/Observador de Estado ==
  data: yh_enc input; vh_obs output; Thm_ref input; whm_0 parameter; titahm_0 parameter; Lh parameter; bh_eq parameter; Jh_eq parameter; rhd parameter; ih parameter; Ts2 parameter; Ms parameter; g parameter
function vh_obs = Observador_Estado_h(yh_enc, Thm_ref, whm_0, titahm_0,...
    Lh, bh_eq, Jh_eq, rhd, ih, Ts2, Ms, g)
    
    % Memorias
    persistent theta_h_obs_prev wh_obs_prev int_e_prev
    
    % Condiciones iniciales
    if isempty(theta_h_obs_prev)
        theta_h_obs_prev = titahm_0;
        wh_obs_prev      = whm_0;    
        int_e_prev       = 0.0; 
    end
    
    % 1. Convertir posición lineal del carro a angular del motor
    theta_h_enc = yh_enc * (2*ih / rhd);
    
    % 2. Error de estimación (Posición real vs observada)
    e_theta_h = theta_h_enc - theta_h_obs_prev;
    
    % 3. Lazo de torque (Física de la planta)
    Torque_net = Thm_ref - (Ms*g*rhd/(2*ih)) - (bh_eq * wh_obs_prev) +...
        (Lh(3) * int_e_prev);
    alpha_phys = Torque_net / Jh_eq; % Aceleración angular
    
    % 4. Derivadas
    dot_wh_obs      = alpha_phys + (Lh(2) * e_theta_h);
    dot_theta_h_obs = wh_obs_prev + (Lh(1) * e_theta_h);

    % 5. Salida del observador
    vh_obs = wh_obs_prev * (rhd / (2*ih));
    
    % 6. Integración Discreta
    theta_h_obs = theta_h_obs_prev + (Ts2 * dot_theta_h_obs);
    wh_obs      = wh_obs_prev      + (Ts2 * dot_wh_obs);
    int_e       = int_e_prev       + (Ts2 * e_theta_h);

    % 7. Actualizar memorias para el siguiente ciclo de reloj
    theta_h_obs_prev = theta_h_obs;
    wh_obs_prev      = wh_obs;
    int_e_prev       = int_e;
end
